simulink model "eval_all"  (R2026a)
settings: Solver=VariableStepAuto  StopTime=1000
undefined symbols (not defined in the file): ekf_param, pf_param, plant_param, r_param, random_seed, u_noise_param
libraries: lib_sensors x6, lib_plant x1
settings Model: Creator=alessandro-nardin  LastModifiedBy=alessandro-nardin
settings RTWCC: Toolchain=Microsoft Visual C++ 2022 v17.0 | nmake (64-bit Windows)

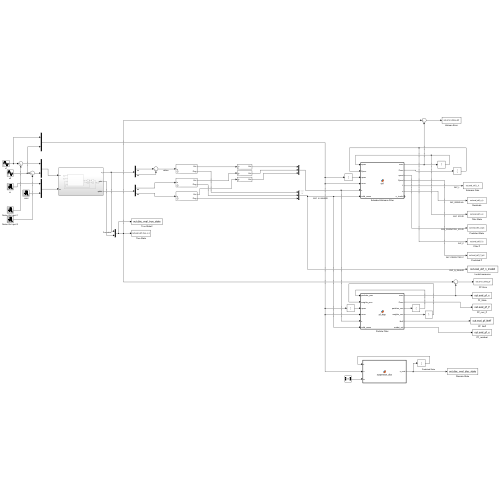
[thumbnail: Simulink's stored preview of the top-level diagram]
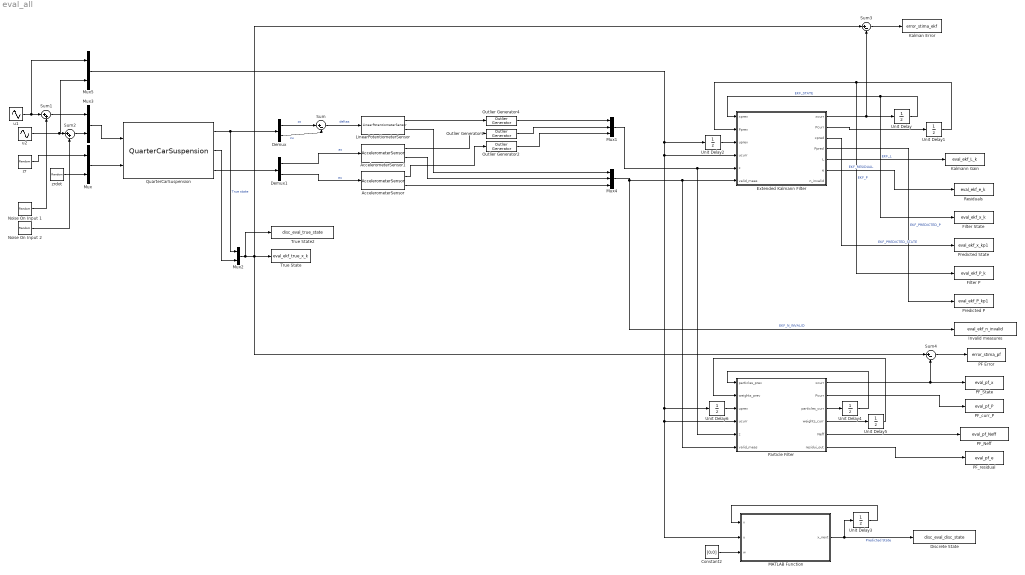
== system eval_all ==
  AccelerometerSensor : lib_sensors/AccelerometerSensor  out_sample_t=ekf_param.sample_t
  AccelerometerSensor1 : lib_sensors/AccelerometerSensor  out_sample_t=ekf_param.sample_t
  Constant2 : Constant  Value=[0;0]
  Demux : Demux  Outputs=2
  Demux1 : Demux  Outputs=2
  Discrete State : ToWorkspace  VariableName=disc_eval_disc_state  SaveFormat=Timeseries  SampleTime=ekf_param.sample_t
  Extended Kalmann Filter : MATLAB Function  TreatAsAtomicUnit=on
  Filter P : ToWorkspace  VariableName=eval_ekf_P_k  SaveFormat=Timeseries  SampleTime=1/ekf_param.freq
  Filter State : ToWorkspace  VariableName=eval_ekf_x_k  SaveFormat=Timeseries  SampleTime=1/ekf_param.freq
  Invalid measures : ToWorkspace  VariableName=eval_ekf_n_invalid  SaveFormat=Timeseries  SampleTime=ekf_param.sample_t
  Kalman Error : ToWorkspace  VariableName=error_stima_ekf  SaveFormat=Timeseries  SampleTime=pf_param.sample_t
  Kalmann Gain : ToWorkspace  VariableName=eval_ekf_L_k  SaveFormat=Timeseries  SampleTime=pf_param.sample_t
  LinearPotentiometerSensor : lib_sensors/LinearPotentiometerSensor  out_sample_t=ekf_param.sample_t
  MATLAB Function : MATLAB Function  TreatAsAtomicUnit=on
  Mux{,2..3,5} (4 alike) : Mux  Inputs=2
  Mux1 : Mux  Inputs=3
  Mux4 : Mux  Inputs=3
  Noise On Input 1 : RandomNumber  Variance=u_noise_param.u1_var  Seed=random_seed+10  SampleTime=0
  Noise On Input 2 : RandomNumber  Variance=u_noise_param.u2_var  Seed=random_seed+10  SampleTime=0
  Outlier Generator1 : lib_sensors/Outlier Generator  outlier_probability=0.002  outlier_amplitude=5  sample_time=acc_param.sample_t
      settings: SourceProductName=Lib Sensors
  Outlier Generator2 : lib_sensors/Outlier Generator  outlier_probability=0.002  outlier_amplitude=5  sample_time=acc_param.sample_t
      settings: SourceProductName=Lib Sensors
  Outlier Generator4 : lib_sensors/Outlier Generator  outlier_probability=0.002  outlier_amplitude=5  sample_time=lpot_param.sample_t
      settings: SourceProductName=Lib Sensors
  PF Error : ToWorkspace  VariableName=error_stima_pf  SaveFormat=Timeseries  SampleTime=pf_param.sample_t
  PF_Neff : ToWorkspace  VariableName=eval_pf_Neff  SaveFormat=Timeseries  SampleTime=-1
  PF_State : ToWorkspace  VariableName=eval_pf_x  SaveFormat=Timeseries  SampleTime=-1
  PF_curr_P : ToWorkspace  VariableName=eval_pf_P  SaveFormat=Timeseries  SampleTime=-1
  PF_residual : ToWorkspace  VariableName=eval_pf_e  SaveFormat=Timeseries  SampleTime=-1
  Particle Filter : MATLAB Function  TreatAsAtomicUnit=on
  Predicted P : ToWorkspace  VariableName=eval_ekf_P_kp1  SaveFormat=Timeseries  SampleTime=1/ekf_param.freq
  Predicted State : ToWorkspace  VariableName=eval_ekf_x_kp1  SaveFormat=Timeseries  SampleTime=1/ekf_param.freq
  QuarterCarSuspension : lib_plant/QuarterCarSuspension  SystemSampleTime=-1  VariantActivationTime=update diagram  EmptyChoice=off  PassThrough=off  PassThroughVariantControl=(default)  EmptyChoiceVariantControl=(default)  AllowFlexibleInterface=on  Latency=0  AutoFrameSizeCalculation=off
      settings: SourceProductName=Lib Plant
  Residuals : ToWorkspace  VariableName=eval_ekf_e_k  SaveFormat=Timeseries  SampleTime=-1
  Sum : Sum  Inputs=|+-
  Sum1 : Sum  Inputs=|++
  Sum2 : Sum  Inputs=|++
  Sum3 : Sum  Inputs=|+-
  Sum4 : Sum  Inputs=|+-
  True State : ToWorkspace  VariableName=eval_ekf_true_x_k  SaveFormat=Timeseries  SampleTime=1/ekf_param.freq
  True State2 : ToWorkspace  VariableName=disc_eval_true_state  SaveFormat=Timeseries  SampleTime=ekf_param.sample_t
  Unit Delay : UnitDelay  InitialCondition=ekf_param.x_init  SampleTime=ekf_param.sample_t
  Unit Delay1 : UnitDelay  InitialCondition=ekf_param.P_init  SampleTime=ekf_param.sample_t
  Unit Delay2 : UnitDelay  InitialCondition=[ 0; 0]  SampleTime=ekf_param.sample_t
  Unit Delay3 : UnitDelay  InitialCondition=[1;0;0;0]  SampleTime=ekf_param.sample_t
  Unit Delay4 : UnitDelay  InitialCondition=pf_param.particles_init  SampleTime=pf_param.sample_t
  Unit Delay5 : UnitDelay  InitialCondition=pf_param.weights_init  SampleTime=pf_param.sample_t
  Unit Delay6 : UnitDelay  InitialCondition=[ 0; 0]  SampleTime=ekf_param.sample_t
  u1 : Sin  Amplitude=943  Frequency=0.5  Phase=0.2  SampleTime=0
  u2 : Sin  Amplitude=2000  Phase=1  SampleTime=0
  zr : RandomNumber  Variance=r_param.rz_var  Seed=random_seed+6  SampleTime=0
  zrdot : RandomNumber  Variance=r_param.rzdot_var  Seed=random_seed+7  SampleTime=0
  wires:
  Demux/1 -> Sum/1  "zs"
  Demux/2 -> Sum/2  "zu"
  Sum/1 -> LinearPotentiometerSensor/1  "deltas"
  Demux1/2 -> AccelerometerSensor/1  "au"
  QuarterCarSuspension/3 -> Demux1/1
  Demux1/1 -> AccelerometerSensor1/1  "as"
  Mux/1 -> QuarterCarSuspension/2
  Extended Kalmann Filter/2(Pcurr) -> Unit Delay1/1
  Unit Delay1/1 -> Extended Kalmann Filter/2(Pprev), Filter P/1  "EKF_P"
  Unit Delay2/1 -> Extended Kalmann Filter/3(uprev)
  AccelerometerSensor1/1 -> Outlier Generator1/1
  Mux1/1 -> Particle Filter/5(z), Extended Kalmann Filter/5(z)
  zrdot/1 -> Mux/2
  Unit Delay/1 -> Extended Kalmann Filter/1(xprev), Filter State/1  "EKF_STATE"
  Extended Kalmann Filter/1(xcurr) -> Sum3/2, Unit Delay/1
  AccelerometerSensor/1 -> Outlier Generator2/1
  Mux4/1 -> Invalid measures/1, Particle Filter/6(valid_meas), Extended Kalmann Filter/6(valid_meas)  "EKF_N_INVALID"
  LinearPotentiometerSensor/2 -> Mux4/1
  AccelerometerSensor1/2 -> Mux4/2
  AccelerometerSensor/2 -> Mux4/3
  LinearPotentiometerSensor/1 -> Outlier Generator4/1
  QuarterCarSuspension/2 -> Mux2/2
  Extended Kalmann Filter/3(xpred) -> Predicted State/1  "EKF_PREDICTED_STATE"
  Extended Kalmann Filter/4(Ppred) -> Predicted P/1  "EKF_PREDICTED_P"
  Extended Kalmann Filter/5(L) -> Kalmann Gain/1  "EKF_L"
  Extended Kalmann Filter/6(e) -> Residuals/1  "EKF_RESIDUAL"
  MATLAB Function/1(x_next) -> Discrete State/1, Unit Delay3/1  "Predicted State"
  Unit Delay3/1 -> MATLAB Function/1(x)
  Constant2/1 -> MATLAB Function/3(w)
  QuarterCarSuspension/1 -> Mux2/1, Demux/1  "True state"
  Mux2/1 -> True State2/1, Sum3/1, Sum4/1, True State/1
  Mux3/1 -> QuarterCarSuspension/1
  Sum1/1 -> Mux3/1
  Sum2/1 -> Mux3/2
  Noise On Input 2/1 -> Sum2/2
  Noise On Input 1/1 -> Sum1/2
  u2/1 -> Mux5/2, Sum2/1
  Outlier Generator4/1 -> Mux1/1
  Outlier Generator1/1 -> Mux1/2
  Outlier Generator2/1 -> Mux1/3
  Unit Delay5/1 -> Particle Filter/2(weights_prev)
  Unit Delay4/1 -> Particle Filter/1(particles_prev)
  Particle Filter/4(weights_curr) -> Unit Delay5/1
  Particle Filter/3(particles_curr) -> Unit Delay4/1
  Mux5/1 -> Unit Delay6/1, Particle Filter/4(ucurr), MATLAB Function/2(u), Extended Kalmann Filter/4(ucurr), Unit Delay2/1
  Unit Delay6/1 -> Particle Filter/3(uprev)
  Particle Filter/2(Pcurr) -> PF_curr_P/1
  Sum3/1 -> Kalman Error/1
  Particle Filter/6(residui_out) -> PF_residual/1
  Particle Filter/5(Neff) -> PF_Neff/1
  Sum4/1 -> PF Error/1
  Particle Filter/1(xcurr) -> Sum4/2, PF_State/1
  zr/1 -> Mux/1
  u1/1 -> Sum1/1, Mux5/1

== matlab function eval_all/MATLAB Function ==
  settings: updateMethod=DISCRETE  sampleTime=ekf_param.sample_t
  data: x input; u input; x_next output size=[ 4 1 ]; w input; plant_param parameter; ekf_param parameter
function x_next = suspension_dics( x, u, w, plant_param, ekf_param)
x_next = suspension_f_dics_euler( x, u, w, plant_param, ekf_param.sample_t);

== matlab function eval_all/Extended Kalmann Filter ==
  settings: updateMethod=DISCRETE  sampleTime=ekf_param.sample_t
  data: xprev input; Pprev input; uprev input; ucurr input; z input; xcurr output size=[ 4 1 ]; Pcurr output; xpred output; Ppred output; plant_param parameter; ekf_param parameter; L output; valid_meas input; e output; n_invalid output
function [ xcurr, Pcurr, xpred, Ppred, L, e, n_invalid ] = ekf( xprev, Pprev, uprev, ucurr, z, plant_param, ekf_param, valid_meas)
[xcurr, Pcurr, xpred, Ppred, L, e, n_invalid] = ekf_step( xprev, Pprev, uprev, ucurr, z, plant_param, ekf_param, valid_meas);

== matlab function eval_all/Particle Filter ==
  settings: updateMethod=DISCRETE  sampleTime=pf_param.sample_t
  data: particles_prev input; weights_prev input; uprev input; ucurr input; z input; plant_param parameter; pf_param parameter; xcurr output; Pcurr output; particles_curr output; weights_curr output; valid_meas input; Neff output; residui_out output
function [xcurr, Pcurr, particles_curr, weights_curr, Neff, residui_out] = pf_step(particles_prev, weights_prev, uprev, ucurr, z, plant_param, pf_param, valid_meas)    % Simulink prenderà plant_param e pf_param direttamente dal workspace
    [xcurr, Pcurr, particles_curr, weights_curr, Neff, residui_out] = pf_step(particles_prev, weights_prev, uprev, ucurr, z, plant_param, pf_param, valid_meas);
end
